simulink model "TorqueVect"  (R2022a)
settings: Solver=VariableStepAuto  StartTime=0.0  StopTime=300  RelTol=1e-3
PreLoadFcn:
  | run('Parameters\FSE_Parameters.m')
values from neighbouring files (symbols this model uses):
  Kd = 0;')    [open_carmaker_gui.m]
  Ki = 0    [open_carmaker_gui.m]
undefined symbols (not defined in the file or in its folder): BRegenEnabledButton, canChannel, CyalphaLookUp, efficiency, Fz_curve, Fz_scaling_long, gearR, izz, jw, kd, ki, Kp, kp, l_f, l_r, lambda, m, Mz_max, N, N_lat, N_long, P_max, pid_kd_lat, pid_kd_long, pid_ki_lat, pid_ki_long, pid_kp_lat, pid_kp_long, R_max, rw, steerR, T_i_max, TC_Decr_Gas, TC_Derivative, TC_Incr_Gas, TC_On, TC_Relay_Off, TC_Relay_On, tireCornerStiffness, Ts, TV_On, TV_Override, velocity_lookup, velocity_lookup_lat, y_ref, yrr_scaling
libraries: simulink x218, slpidlib x135, CarMaker4SL x73, TractionControlLibrary x13, canmsglib x9, canlib x8, TorqueVectoringLibrary x6, simulink_extras x4, PedalConversionLibrary x3, PowerControlLibrary x1
(part 26 of 26)

== system TorqueVect/CarMaker/IPG Vehicle/PowerTrain/PTControl Example/PTControl_TV_MFE3/New TC/TC R3/traction_controller/traction_controller/PD Controller ==
  dslip : Inport
  enable_tc : Inport  Port=2
  Kp : Inport  Port=3
  Kd : Inport  Port=4
  if_not_on_target : ActionPort
  Constant : Constant  Value=100
  PID Controller : slpidlib/PID Controller  Controller=PD  Form=Parallel  TimeDomain=Continuous-time  UseExternalTs=off  SampleTime=-1  IntegratorMethod=Forward Euler  FilterMethod=Forward Euler  ControllerParametersSource=external  P=Kp  I=Ki  UseKiTs=off  D=Kd  N=100  UseFilter=on  TunerSelectOption=Transfer Function Based (PID Tuner App)  InitialConditionSource=internal  InitialConditionForIntegrator=0  InitialConditionForFilter=0  DifferentiatorICPrevScaledInput=0  ExternalReset=none  TrackingMode=off  Kt=1  LimitOutput=on  SatLimitsSource=internal  UpperSaturationLimit=240  LowerSaturationLimit=0  LinearizeAsGain=on  AntiWindupMode=none  Kb=1  POutMin=[]  POutMax=[]  IOutMin=[]  IOutMax=[]  DOutMin=[]  DOutMax=[]  NOutMin=[]  NOutMax=[]  SumOutMin=[]  SumOutMax=[]  SaturationOutMin=[]  SaturationOutMax=[]  PParamMin=[]  PParamMax=[]  IParamMin=[]  IParamMax=[]  DParamMin=[]  DParamMax=[]  NParamMin=[]  NParamMax=[]  KbParamMin=[]  KbParamMax=[]  KtParamMin=[]  KtParamMax=[]  KbOutMin=[]  KbOutMax=[]  KtOutMin=[]  KtOutMax=[]  IntegratorOutMin=[]  IntegratorOutMax=[]  FilterOutMin=[]  FilterOutMax=[]  SumI1OutMin=[]  SumI1OutMax=[]  SumI2OutMin=[]  SumI2OutMax=[]  SumI3OutMin=[]  SumI3OutMax=[]  SumI4OutMin=[]  SumI4OutMax=[]  SumDOutMin=[]  SumDOutMax=[]  DifferentiatorOutMin=[]  DifferentiatorOutMax=[]  FilterDiffOutCoefMin=[]  FilterDiffOutCoefMax=[]  ReciprocalOutMin=[]  ReciprocalOutMax=[]  SumDenOutMin=[]  SumDenOutMax=[]  SumNumOutMin=[]  SumNumOutMax=[]  DivideOutMin=[]  DivideOutMax=[]  UdiffTsProdOutMin=[]  UdiffTsProdOutMax=[]  NTsProdOutMin=[]  NTsProdOutMax=[]  UintegralTsProdOutMin=[]  UintegralTsProdOutMax=[]  UngainTsProdOutMin=[]  UngainTsProdOutMax=[]  ClampingZeroOutDataTypeStr=Inherit: Inherit via back propagation  ClampingZeroOutMin=[]  ClampingZeroOutMax=[]  FilterDenConstantOutDataTypeStr=Inherit: Inherit via back propagation  FilterDenConstantOutMin=[]  FilterDenConstantOutMax=[]  PCopyOutDataTypeStr=Inherit: Inherit via back propagation  PCopyOutMin=[]  PCopyOutMax=[]  NCopyOutDataTypeStr=Inherit: Inherit via back propagation  NCopyOutMin=[]  NCopyOutMax=[]  IntegratorContinuousStateAttributes=''  IntegratorStateMustResolveToSignalObject=off  IntegratorRTWStateStorageClass=Auto  FilterContinuousStateAttributes=''  FilterStateMustResolveToSignalObject=off  FilterRTWStateStorageClass=Auto  ParallelPVariant=ExternalParameters  IdealPVariant=Disabled  IVariant=Disabled  DVariant=ExternalParameters  IntegratorVariant=Disabled  SatVariant=Enabled  AWVariant=Disabled  PCopyVariant=Disabled  TRVariant=Disabled  FdbkBlocksVariant=Forward  IdealPFdbkVariant=Disabled  SatFdbkVariant=Disabled  DerivativeFilterVariant=ContFilter  NVariant=ExternalParameters  NCopyVariant=Disabled  FilterICVariant=InternalICsFilter  IntegratorICVariant=Disabled  ExternalResetVariant=Disabled  TRSumVariant=Passthrough  SumFdbkVariant=Disabled  SumVariant=Sum_PD  TsampFilterVariant=InternalTs  TsampNgainVariant=Passthrough  TsampIntegralVariant=Disabled_SignalSpec  ExternalSaturationOutDataTypeStr=Inherit: Same as second input  aMode=0
  Product : Product
  Saturation : Saturate  UpperLimit=1  LowerLimit=0  OutDataTypeStr=uint8
  delta_torque : Outport  VectorParamsAs1DForOutWhenUnconnected=off
  wires:
  Kp/1 -> PID Controller/2
  enable_tc/1 -> Saturation/1
  PID Controller/1 -> Product/1
  Saturation/1 -> Product/2
  Product/1 -> delta_torque/1
  Kd/1 -> PID Controller/3
  Constant/1 -> PID Controller/4
  dslip/1 -> PID Controller/1

== system TorqueVect/CarMaker/IPG Vehicle/PowerTrain/PTControl Example/PTControl_TV_MFE3/New TC/TC R3/traction_controller/traction_controller/default ==
  if_on_target : ActionPort
  Constant : Constant  Value=0
  no_change : Outport  VectorParamsAs1DForOutWhenUnconnected=off
  wires:
  Constant/1 -> no_change/1

== system TorqueVect/CarMaker/IPG Vehicle/PowerTrain/PTControl Example/PTControl_TV_MFE3/New TC/TC R4/traction_controller/traction_controller/PD Controller ==
  dslip : Inport
  enable_tc : Inport  Port=2
  Kp : Inport  Port=3
  Kd : Inport  Port=4
  if_not_on_target : ActionPort
  Constant : Constant  Value=100
  PID Controller : slpidlib/PID Controller  Controller=PD  Form=Parallel  TimeDomain=Continuous-time  UseExternalTs=off  SampleTime=-1  IntegratorMethod=Forward Euler  FilterMethod=Forward Euler  ControllerParametersSource=external  P=Kp  I=Ki  UseKiTs=off  D=Kd  N=100  UseFilter=on  TunerSelectOption=Transfer Function Based (PID Tuner App)  InitialConditionSource=internal  InitialConditionForIntegrator=0  InitialConditionForFilter=0  DifferentiatorICPrevScaledInput=0  ExternalReset=none  TrackingMode=off  Kt=1  LimitOutput=on  SatLimitsSource=internal  UpperSaturationLimit=240  LowerSaturationLimit=0  LinearizeAsGain=on  AntiWindupMode=none  Kb=1  POutMin=[]  POutMax=[]  IOutMin=[]  IOutMax=[]  DOutMin=[]  DOutMax=[]  NOutMin=[]  NOutMax=[]  SumOutMin=[]  SumOutMax=[]  SaturationOutMin=[]  SaturationOutMax=[]  PParamMin=[]  PParamMax=[]  IParamMin=[]  IParamMax=[]  DParamMin=[]  DParamMax=[]  NParamMin=[]  NParamMax=[]  KbParamMin=[]  KbParamMax=[]  KtParamMin=[]  KtParamMax=[]  KbOutMin=[]  KbOutMax=[]  KtOutMin=[]  KtOutMax=[]  IntegratorOutMin=[]  IntegratorOutMax=[]  FilterOutMin=[]  FilterOutMax=[]  SumI1OutMin=[]  SumI1OutMax=[]  SumI2OutMin=[]  SumI2OutMax=[]  SumI3OutMin=[]  SumI3OutMax=[]  SumI4OutMin=[]  SumI4OutMax=[]  SumDOutMin=[]  SumDOutMax=[]  DifferentiatorOutMin=[]  DifferentiatorOutMax=[]  FilterDiffOutCoefMin=[]  FilterDiffOutCoefMax=[]  ReciprocalOutMin=[]  ReciprocalOutMax=[]  SumDenOutMin=[]  SumDenOutMax=[]  SumNumOutMin=[]  SumNumOutMax=[]  DivideOutMin=[]  DivideOutMax=[]  UdiffTsProdOutMin=[]  UdiffTsProdOutMax=[]  NTsProdOutMin=[]  NTsProdOutMax=[]  UintegralTsProdOutMin=[]  UintegralTsProdOutMax=[]  UngainTsProdOutMin=[]  UngainTsProdOutMax=[]  ClampingZeroOutDataTypeStr=Inherit: Inherit via back propagation  ClampingZeroOutMin=[]  ClampingZeroOutMax=[]  FilterDenConstantOutDataTypeStr=Inherit: Inherit via back propagation  FilterDenConstantOutMin=[]  FilterDenConstantOutMax=[]  PCopyOutDataTypeStr=Inherit: Inherit via back propagation  PCopyOutMin=[]  PCopyOutMax=[]  NCopyOutDataTypeStr=Inherit: Inherit via back propagation  NCopyOutMin=[]  NCopyOutMax=[]  IntegratorContinuousStateAttributes=''  IntegratorStateMustResolveToSignalObject=off  IntegratorRTWStateStorageClass=Auto  FilterContinuousStateAttributes=''  FilterStateMustResolveToSignalObject=off  FilterRTWStateStorageClass=Auto  ParallelPVariant=ExternalParameters  IdealPVariant=Disabled  IVariant=Disabled  DVariant=ExternalParameters  IntegratorVariant=Disabled  SatVariant=Enabled  AWVariant=Disabled  PCopyVariant=Disabled  TRVariant=Disabled  FdbkBlocksVariant=Forward  IdealPFdbkVariant=Disabled  SatFdbkVariant=Disabled  DerivativeFilterVariant=ContFilter  NVariant=ExternalParameters  NCopyVariant=Disabled  FilterICVariant=InternalICsFilter  IntegratorICVariant=Disabled  ExternalResetVariant=Disabled  TRSumVariant=Passthrough  SumFdbkVariant=Disabled  SumVariant=Sum_PD  TsampFilterVariant=InternalTs  TsampNgainVariant=Passthrough  TsampIntegralVariant=Disabled_SignalSpec  ExternalSaturationOutDataTypeStr=Inherit: Same as second input  aMode=0
  Product : Product
  Saturation : Saturate  UpperLimit=1  LowerLimit=0  OutDataTypeStr=uint8
  delta_torque : Outport  VectorParamsAs1DForOutWhenUnconnected=off
  wires:
  Kp/1 -> PID Controller/2
  enable_tc/1 -> Saturation/1
  PID Controller/1 -> Product/1
  Saturation/1 -> Product/2
  Product/1 -> delta_torque/1
  Kd/1 -> PID Controller/3
  Constant/1 -> PID Controller/4
  dslip/1 -> PID Controller/1

== system TorqueVect/CarMaker/IPG Vehicle/PowerTrain/PTControl Example/PTControl_TV_MFE3/New TC/TC R4/traction_controller/traction_controller/default ==
  if_on_target : ActionPort
  Constant : Constant  Value=0
  no_change : Outport  VectorParamsAs1DForOutWhenUnconnected=off
  wires:
  Constant/1 -> no_change/1

== matlab function TorqueVect/CarMaker/IPG Vehicle/PowerTrain/PTControl Example/PTControl_TV_MFE25/Full Control Loop/Reference Generator/Y_Reference ==
  data: target_kappa input; vehicle_speed input; y_ref1 output; min_speed input; y_ref2 output; y_ref3 output; y_ref4 output
function [y_ref1,y_ref2, y_ref3, y_ref4] = Y_Reference( target_kappa,  vehicle_speed,min_speed)

%min_speed = 0.1;
y_ref = ones(4,1).*target_kappa;

if vehicle_speed <= min_speed %arbirtary, just need something otherwise car won't start. Should look into its impact
    for i = 1:4
        y_ref(i) = min_speed*target_kappa(i);
        disp(vehicle_speed)
    end

else
    for i = 1:4
        y_ref(i) = vehicle_speed*target_kappa(i);
        disp(vehicle_speed)
    end
end
y_ref1=y_ref(1);
y_ref2=y_ref(2);
y_ref3=y_ref(3);
y_ref4=y_ref(4);

== matlab function TorqueVect/CarMaker/IPG Vehicle/PowerTrain/PTControl Example/PTControl_TV_MFE25/Full Control Loop/Torque Allocation ==
  data: F input size=[1 4]; u input size=1; omega input size=[1 4]; u1 output size=1; u2 output size=1; u3 output size=1; u4 output size=1; P_max input; T_i_max input; lamda input
function [u1, u2, u3, u4] = fcn(F, u, omega, P_max, T_i_max, lamda)
    n       = 4;            % four wheels
    %P_max   = 80000;          % W, power cap
    %T_i_max = 21;           % Nm, max torque of each wheel
    T_max   = n * T_i_max;  % Total max torque

    % If we have any negative or zero value, the objective becomes ill
    % defined, add check 
    % If load on tire is smaller than 100, assume wrong and set to standard
    % value of 500
    F(F < 100) = 500;
      

    % Define cost function
    F_total = sum(F);

    w = sqrt(F_total ./ F);
    D = diag(w);                % Weighted penalty matrix
    A = ones(1, n);             % Converted torque equality constraint
    b = u * T_max;
    %lamda = 0.5;                % Scaling factor

    fun = @(x) norm(b - A*x) + lamda*norm(D*x);

    % Define inequality constraints to satisfy power cap
    A_ineq = omega*13.39;
    b_ineq = P_max;

   
    % Define bounds on solution, x = [4x1]
    ub = T_i_max * ones(n, 1);
    lb = zeros(n, 1);

    % Solve the optimization problem
    x0 = zeros(n, 1);
    opts = optimoptions('fmincon','Algorithm','sqp');
    x = fmincon(fun,x0,A_ineq,b_ineq,[],[],lb,ub,[],opts);

    %% Export Solution
    u1 = x(1);
    u2 = x(2);
    u3 = x(3);
    u4 = x(4);
end

== matlab function TorqueVect/CarMaker/IPG Vehicle/PowerTrain/PTControl Example/PTControl_ALL_CTRL_VC_REGEN/Subsystem1/TorqueSplit/MATLAB Function ==
  data: f_in input; fl_out output; r_in input; fr_out output; rl_out output; rr_out output; maxTrq input
function [fl_out, fr_out, rl_out, rr_out]= fcn(f_in, r_in, maxTrq)

front = f_in * 0.5;
rear = r_in * 0.5;

%% Convert for regen
if f_in < 0
    front = front * -1;
    rear = rear * -1;
end

%% Check for > maxTrq
if front > maxTrq && rear > maxTrq
    front = maxTrq;
    rear = maxTrq;
elseif front > maxTrq
    rear = rear + (front-maxTrq);
    front = maxTrq;
elseif rear > maxTrq
    front = front + (rear-maxTrq);
    rear = maxTrq;
end

%% Convert back for regen
if f_in < 0
    front = front * -1;
    rear = rear * -1;
end

fl_out = front;
fr_out = front;
rl_out = rear;
rr_out = rear;

== matlab function TorqueVect/CarMaker/IPG Vehicle/PowerTrain/PTControl Example/PTControl_TV_MFE25/Full Control Loop/MATLAB Function ==
  data: F input; u input; u1 output; omega input; P_max input; T_i_max input; lamda input; u2 output; u3 output; u4 output
function [u1, u2, u3, u4] = fcn(F, u, omega, P_max, T_i_max, lamda)
    n       = 4;            % four wheels
    %P_max   = 80000;          % W, power cap
    %T_i_max = 21;           % Nm, max torque of each wheel
    T_max   = n * T_i_max;  % Total max torque

    % If we have any negative or zero value, the objective becomes ill
    % defined, add check 
    % If load on tire is smaller than 100, assume wrong and set to standard
    % value of 500
    F(F < 100) = 500;
      

    % Define cost function
    F_total = sum(F);

    w = sqrt(F_total ./ F);
    D = diag(w);                % Weighted penalty matrix
    A = ones(1, n);             % Converted torque equality constraint
    b = u * T_max;
    %lamda = 0.5;                % Scaling factor

    fun = @(x) norm(b - A*x) + lamda*norm(D*x);

    % Define inequality constraints to satisfy power cap
    A_ineq = omega' * 13.39;
    b_ineq = P_max;

   
    % Define bounds on solution, x = [4x1]
    ub = T_i_max * ones(n, 1);
    lb = zeros(n, 1);                                                                                                                                                                                                                                                                                                                                                                                                                                                                                                                                                                                                                                                                                                                                                                                                                                                                                                                                                                                                                                                                                                                                                                                                                                                                                                                                                                                                                                                                                                                                                                                         

    % Solve the optimization problem                                                                                                                                                                                                                                                                                                                                                                                                                                                                                                                                                                                                                                                                                                                                                                                                                                                                                                                                                                                                                                                                                                                                                    
    x0 = zeros(n, 1);
    opts = optimoptions('fmincon','Algorithm','sqp');
    x = fmincon(fun,x0,A_ineq,b_ineq,[],[],lb,ub,[],opts);

    %% Export Solution
    u1 = x(1);
    u2 = x(2);
    u3 = x(3);
    u4 = x(4);                  
end

== matlab function TorqueVect/CarMaker/IPG Vehicle/PowerTrain/PTControl Example/PTControl_TV_MFE2/Subsystem/TorqueSplit/MATLAB Function ==
  data: f_in input; fl_out output; r_in input; fr_out output; rl_out output; rr_out output; maxTrq input
function [fl_out, fr_out, rl_out, rr_out]= fcn(f_in, r_in, maxTrq)

front = f_in * 0.5;
rear = r_in * 0.5;

%% Convert for regen
if f_in < 0
    front = front * -1;
    rear = rear * -1;
end

%% Check for > maxTrq
if front > maxTrq && rear > maxTrq
    front = maxTrq;
    rear = maxTrq;
elseif front > maxTrq
    rear = rear + (front-maxTrq);
    front = maxTrq;
elseif rear > maxTrq
    front = front + (rear-maxTrq);
    rear = maxTrq;
end

%% Convert back for regen
if f_in < 0
    front = front * -1;
    rear = rear * -1;
end

fl_out = front;
fr_out = front;
rl_out = rear;
rr_out = rear;

== matlab function TorqueVect/CarMaker/IPG Vehicle/PowerTrain/PTControl Example/PTControl_TV_MFE3/Full Control Loop/MATLAB Function ==
  data: F input; u input; u1 output; omega input; P_max input; T_i_max input; lamda input; u2 output; u3 output; u4 output
function [u1, u2, u3, u4] = fcn(F, u, omega, P_max, T_i_max, lamda)
    n       = 4;            % four wheels
    %P_max   = 80000;          % W, power cap
    %T_i_max = 21;           % Nm, max torque of each wheel
    T_max   = n * T_i_max;  % Total max torque

    % If we have any negative or zero value, the objective becomes ill
    % defined, add check 
    % If load on tire is smaller than 100, assume wrong and set to standard
    % value of 500
%     F(F < 100) = 500;
      

    % Define cost function
    F_total = sum(F);

    w = sqrt(F_total ./ F);
    D = diag(w);                % Weighted penalty matrix
    A = ones(1, n);             % Converted torque equality constraint
    b = u * T_max;
    %lamda = 0.5;                % Scaling factor

    fun = @(x) norm(b - A*x) + lamda*norm(D*x);

    % Define inequality constraints to satisfy power cap
    A_ineq = omega*13.39;
    b_ineq = P_max;

   
    % Define bounds on solution, x = [4x1]
    ub = T_i_max * ones(n, 1);
    lb = zeros(n, 1);                                                                                                                                                                                                                                                                                                                                                                                                                                                                                                                                                                                                                                                                                                                                                                                                                                                                                                                                                                                                                                                                                                                                                                                                                                                                                                                                                                                                                                                                                                                                                                                         

    % Solve the optimization problem                                                                                                                                                                                                                                                                                                                                                                                                                                                                                                                                                                                                                                                                                                                                                                                                                                                                                                                                                                                                                                                                                                                                                    
    x0 = zeros(n, 1);
    opts = optimoptions('fmincon','Algorithm','sqp');
    x = fmincon(fun,x0,A_ineq,b_ineq,[],[],lb,ub,[],opts);

    %% Export Solution
    u1 = x(1);
    u2 = x(2);
    u3 = x(3);
    u4 = x(4);                  
end

== matlab function TorqueVect/CarMaker/IPG Vehicle/PowerTrain/PTControl Example/PTControl_TV_MFE3/Full Control Loop/Reference Generator/Y_Reference ==
  data: target_kappa input; vehicle_speed input; y_ref1 output; min_speed input; y_ref2 output; y_ref3 output; y_ref4 output
function [y_ref1,y_ref2, y_ref3, y_ref4] = Y_Reference( target_kappa,  vehicle_speed,min_speed)

%min_speed = 0.1;
y_ref = ones(4,1).*target_kappa;

if vehicle_speed <= min_speed %arbirtary, just need something otherwise car won't start. Should look into its impact
    for i = 1:4
        y_ref(i) = min_speed*target_kappa(i);
        disp(vehicle_speed)
    end

else
    for i = 1:4
        y_ref(i) = vehicle_speed*target_kappa(i);
        disp(vehicle_speed)
    end
end
y_ref1=y_ref(1);
y_ref2=y_ref(2);
y_ref3=y_ref(3);
y_ref4=y_ref(4);

== matlab function TorqueVect/CarMaker/IPG Vehicle/PowerTrain/PTControl Example/PTControl_TV_MFE3/Full Control Loop/Torque Allocation ==
  data: F input size=[1 4]; u input size=1; omega input size=[1 4]; u1 output size=1; u2 output size=1; u3 output size=1; u4 output size=1; P_max input; T_i_max input; lamda input
function [u1, u2, u3, u4] = fcn(F, u, omega, P_max, T_i_max, lamda)
    n       = 4;            % four wheels
    %P_max   = 80000;          % W, power cap
    %T_i_max = 21;           % Nm, max torque of each wheel
    T_max   = n * T_i_max;  % Total max torque

    % If we have any negative or zero value, the objective becomes ill
    % defined, add check 
    % If load on tire is smaller than 100, assume wrong and set to standard
    % value of 500
    F(F < 100) = 500;
      

    % Define cost function
    F_total = sum(F);

    w = sqrt(F_total ./ F);
    D = diag(w);                % Weighted penalty matrix
    A = ones(1, n);             % Converted torque equality constraint
    b = u * T_max;
    %lamda = 0.5;                % Scaling factor

    fun = @(x) norm(b - A*x) + lamda*norm(D*x);

    % Define inequality constraints to satisfy power cap
    A_ineq = omega*13.39;
    b_ineq = P_max;

   
    % Define bounds on solution, x = [4x1]
    ub = T_i_max * ones(n, 1);
    lb = zeros(n, 1);

    % Solve the optimization problem
    x0 = zeros(n, 1);
    opts = optimoptions('fmincon','Algorithm','sqp');
    x = fmincon(fun,x0,A_ineq,b_ineq,[],[],lb,ub,[],opts);

    %% Export Solution
    u1 = x(1);
    u2 = x(2);
    u3 = x(3);
    u4 = x(4);
end

== matlab function TorqueVect/CarMaker/IPG Vehicle/PowerTrain/PTControl Example/PTControl_ALL_CTRL_VC_REGEN/Subsystem/TorqueSplit/MATLAB Function ==
  data: f_in input; fl_out output; r_in input; fr_out output; rl_out output; rr_out output; maxTrq input
function [fl_out, fr_out, rl_out, rr_out]= fcn(f_in, r_in, maxTrq)

front = f_in * 0.5;
rear = r_in * 0.5;

%% Convert for regen
if f_in < 0
    front = front * -1;
    rear = rear * -1;
end

%% Check for > maxTrq
if front > maxTrq && rear > maxTrq
    front = maxTrq;
    rear = maxTrq;
elseif front > maxTrq
    rear = rear + (front-maxTrq);
    front = maxTrq;
elseif rear > maxTrq
    front = front + (rear-maxTrq);
    rear = maxTrq;
end

%% Convert back for regen
if f_in < 0
    front = front * -1;
    rear = rear * -1;
end

fl_out = front;
fr_out = front;
rl_out = rear;
rr_out = rear;

== matlab function TorqueVect/CarMaker/IPG Vehicle/PowerTrain/PTControl Example/PTControl_ALL_CTRL_VC_MFE24/Subsystem/TorqueSplit/MATLAB Function ==
  data: f_in input; fl_out output; r_in input; fr_out output; rl_out output; rr_out output; maxTrq input
function [fl_out, fr_out, rl_out, rr_out]= fcn(f_in, r_in, maxTrq)

front = f_in * 0.5;
rear = r_in * 0.5;

%% Convert for regen
if f_in < 0
    front = front * -1;
    rear = rear * -1;
end

%% Check for > maxTrq
if front > maxTrq && rear > maxTrq
    front = maxTrq;
    rear = maxTrq;
elseif front > maxTrq
    rear = rear + (front-maxTrq);
    front = maxTrq;
elseif rear > maxTrq
    front = front + (rear-maxTrq);
    rear = maxTrq;
end

%% Convert back for regen
if f_in < 0
    front = front * -1;
    rear = rear * -1;
end

fl_out = front;
fr_out = front;
rl_out = rear;
rr_out = rear;
